simulink model "untitled"  (R2017a)
settings: Solver=VariableStepAuto  StartTime=0.0  StopTime=10.0  RelTol=1e-3
settings Model: Creator=leoap  LastModifiedBy=leoap

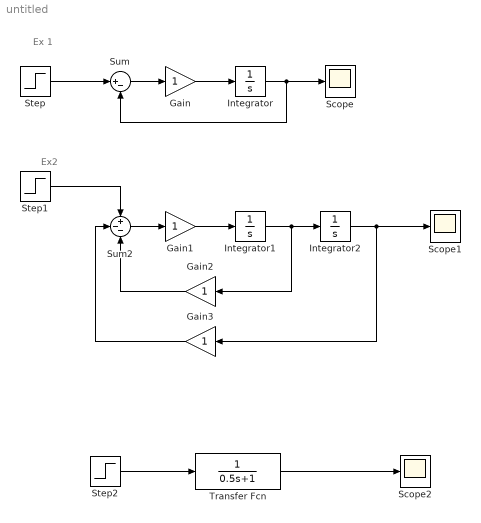
== system untitled ==
  note: Ex2
  note: Ex 1
  Gain{,1..3} (4 alike) : Gain
  Integrator : Integrator
  Integrator1 : Integrator
  Integrator2 : Integrator
  Scope : Scope
  Scope1 : Scope
  Scope2 : Scope
  Step : Step  SampleTime=0
  Step1 : Step  SampleTime=0
  Step2 : Step  SampleTime=0
  Sum : Sum  Inputs=|+-
  Sum2 : Sum  Inputs=+--
  Transfer Fcn : TransferFcn  Denominator=[0.5 1]
  wires:
  Gain/1 -> Integrator/1
  Sum/1 -> Gain/1
  Integrator/1 -> Sum/2, Scope/1
  Step/1 -> Sum/1
  Integrator1/1 -> Gain2/1, Integrator2/1
  Gain1/1 -> Integrator1/1
  Step1/1 -> Sum2/1
  Sum2/1 -> Gain1/1
  Integrator2/1 -> Gain3/1, Scope1/1
  Gain2/1 -> Sum2/3
  Gain3/1 -> Sum2/2
  Transfer Fcn/1 -> Scope2/1
  Step2/1 -> Transfer Fcn/1
